simulink model "GreenCraneActualPrints"  (R2025b)
settings: Solver=VariableStepAuto  StartTime=0.0  StopTime=30  RelTol=1e-3
model workspace (MATLAB code in the model file):
  | clear;
  | %% Hydraulics
  | 
  | %Liquid
  | rho = 875;
  | beta = 1000; %MPa
  | 
  | %Pump
  | pP = 10e6; %100 bar i pascal, velger den sjøl med å skru
  | 
  | %Initial pA_Cyl
  | pA_Cyl_Initial = 67;    %Bar
  | 
  | %-------------------DCV-----------------------
  | dp0 = 20e5; %Nominal pressure drop, Pa
  | Q0 = 18/6e4; %Nominal flow, m^3/s
  | Cd = 0.55; %Discharge coefficient
  | AdMax_SI = Q0/(Cd*(2/rho*dp0)^0.5); %Discharge area m^2
  | AdMax = AdMax_SI*1e6;
  | 
  | Tau_DCV = 0.1; % [s] foreløbig
  | 
  | %TauP = 0.322; % Tau for pressure lowpass filter 49Hz veldig kraftig det fra Twincat
  | TauP = 1/(2*pi*5); % 5hz
  | %% DCV Orifice Area Vectors
  | 
  | % Deadband control signal thresholds
  | u_dead_up    = 0.236;
  | u_dead_down  = 0.206;
  | 
  | % Spool position at deadband
  | spool_dead_up   = 1.1182 * u_dead_up   - 0.0325;
  | spool_dead_down = 1.1075 * u_dead_down - 0.0416;
  | 
  | % Polynomial: spool position as function of Kv [L/min/sqrt(bar)]
  | % Valid from u = 0.25 to max stroke
  | p_spool_of_Kv_up   = [0.0018653, -0.033672,  0.22033, -0.65618,  0.83411, -0.047269, 0.26252];
  | p_spool_of_Kv_down = [0.00098272, -0.017507,  0.11599, -0.34851,  0.41222,  0.17643,  0.2076];
  | 
  | % Linear model slopes: spool_pos = spool_dead + slope * Kv
  | slope_Kv_up   = 0.3410;
  | slope_Kv_down = 0.4248;
  | 
  | % Evaluate polynomial over valid Kv range
  | Kv_range   = linspace(0.09, 4, 10000);
  | spool_up   = polyval(p_spool_of_Kv_up,   Kv_range);
  | spool_down = polyval(p_spool_of_Kv_down, Kv_range);
  | 
  | % Breakpoints: u = 0.25 to 0.50 in steps of 0.05, then max
  | u_breakpoints = 0.25:0.05:1.0;
  | 
  | % Corresponding spool positions
  | spool_bp_up   = 1.1182 * u_breakpoints - 0.0325;
  | spool_bp_down = 1.1075 * u_breakpoints - 0.0416;
  | 
  | % Find Kv at each breakpoint using nearest-index lookup
  | Kv_bp_up   = zeros(1, length(u_breakpoints));
  | Kv_bp_down = zeros(1, length(u_breakpoints));
  | for i = 1:length(u_breakpoints)
  |     if u_breakpoints(i) <= 0.25
  |         % Use linear model for transition point
  |         Kv_bp_up(i)   = (spool_bp_up(i)   - spool_dead_up)   / slope_Kv_up;
  |         Kv_bp_down(i) = (spool_bp_down(i) - spool_dead_down) / slope_Kv_down;
  |     else
  |         % Use polynomial inversion via nearest-index lookup
  |         [~, idx_up]   = min(abs(spool_up   - spool_bp_up(i)));
  |         [~, idx_down] = min(abs(spool_down - spool_bp_down(i)));
  |         Kv_bp_up(i)   = Kv_range(idx_up);
  |         Kv_bp_down(i) = Kv_range(idx_down);
  |     end
  | end
  | 
  | % Kv at max spool
  | [~, idx_max_up]   = max(spool_up);
  | [~, idx_max_down] = max(spool_down);
  | Kv_max_up   = Kv_range(idx_max_up);
  | Kv_max_down = Kv_range(idx_max_down);
  | 
  | % Unit conversion: L/min/sqrt(bar) -> m³/s/sqrt(Pa)
  | Kv_unit_conv = sqrt(1e-5) / 6e4;
  | 
  | % Convert all Kv breakpoints to area [m²]
  | A_bp_up   = (Kv_bp_up   * Kv_unit_conv) / (Cd * sqrt(2/rho));
  | A_bp_down = (Kv_bp_down * Kv_unit_conv) / (Cd * sqrt(2/rho));
  | A_max_up  = (Kv_max_up  * Kv_unit_conv) / (Cd * sqrt(2/rho));
  | A_max_down= (Kv_max_down* Kv_unit_conv) / (Cd * sqrt(2/rho));
  | 
  | % Orifice area vectors [m²]: [leakage, crack-open, u=0.30...0.50, fully-open]
  | orifice_area_up   = [1e-9, A_bp_up,   A_max_up];
  | orifice_area_down = [1e-9, A_bp_down, A_max_down];
  | 
  | % Control member position vectors (must match area vectors one-to-one)
  | u_max_pos = 1.05; % position for max area point, beyond valid range to avoid duplicate
  | % control_pos_up   = [0, u_breakpoints, u_max_pos];
  | % control_pos_down = [0, u_breakpoints, u_max_pos]; Nye under
  | 
  | control_pos_up   = [0, spool_bp_up,   1.1182 * u_max_pos - 0.0325];
  | control_pos_down = [0, spool_bp_down, 1.1075 * u_max_pos - 0.0416];
  | 
  | % ------------------CBV-------------------
  | alpha = 5; %Pilot ratio
  | pCr_A = 230e5; %Pa.
  | dp_open_A = 150e5; %Pa setter lik pcrack først
  | 
  | Cd_CBV = 0.8;
  | AdMax_CBV = (60 / 6e4) / sqrt(2/rho * 16e5) / Cd_CBV; %SJekk over denne
  | 
  | %-----------------Cylinder-----------------
  | d = 65; %mm
  | dr = 35; %mm
  | A = pi*d^2/4; %mm^2
  | Ar = pi*dr^2/4;  %mm^2
  | Aa = A - Ar; %mm^2
  | h = 500; %mm slaglengde
  | L0 = 272; %mm , dødlengde
  | dx = 0; %Dummy mm dx er mellom 0 og 500mm
  | L = h + L0 + dx; %mm variable length eller initial pos
  | 
  | %Weight (bruker ikke lenger?)
  | m = 75*4 + 20 + 90; %kg
  | g = 9.81; %m/s^2
  | MG = m*g; %Force from weight
  | 
  | %inital postition
  | x_Init = 100; %mm
  | 
  | 
  | %% Geometric properties
  | 
  | % Cylinder Translation lower hinge
  | Cx = 427; %mm translation from global coordinate
  | Cz = -1057; %mm translation
  | 
  | % Crane arm
  | theta_Init = 73.04- 90; %deg når kran er nede
  | thetaDot_Init = 0;
  | L1 = 3680; %mm length of beam
  | B1 = 100; %mm width of beam
  | H1 = 150; %mm height
  | t1 = 6; %mm thickness
  | revBasePinDia = 60; %mm of the pin in the main hinge
  | revBasePinLength = 185.5; %mm of the pin in the main hinge
  | 
  | %Cylinder
  | rEar = 35; %mm radius of the bearing ear
  | tEar = 30; %mm thickness of ear
  | earToCylTop = 52.45; %mm center of ear to top of cylinder in bottom pos
  | earToCylBot = 40.62; %mm center of ear to bottom cylinder in bottom pos
  | cylDia = 75; %mm Diameter of cylinger housing
  | cylLength = 682; %mm length of housing
  | rodLength = 565.26; %mm length of rod
  | rodDia = 35; %mm rod diameter
  | rodToCyl = 132; %mm Length in bottom pos from bottom of cylinder to bottom of rod without rod plate
  | revCylPinDia = 25; %mm diameter of the pin that the bearing of the top and bottom of cylinder revolves around
  | revCylPinLength = 84; %mm length of the pin
  | rPiston = 65/2; %mm radius of piston
  | tPiston = 40; %mm thickness of piston
  | 
  | %Ear top from global coordinate system
  | abx = 564.99; %mm; in the bottom pos
  | aby = 133; %mm in the bottom pos
  | 
  | % PayLoad
  | L2 = 210; %mm of the whole weight block
  | B2 = 700; %mm
  | H2 = 300; %mm
  | dY_PL_Beam = 75; %mm center of beam to center of payload
  | 
  | %% Mass properties (mass and center of mass)
  | beam_mass = 415.740; %kg mass of payload and beam
  | beam_COM = [3216.15, 61.48, 0.00]; %mm Old value x=3013.15mm
  | 
  | cyl_house_mass = 10.46699; %kg
  | cyl_house_COM = [260.99, 0.16, 0.00]; %mm from center of lowerjoint coordinate system
  | 
  | cyl_rod_mass = 4.81658; %kg mass of cylinder rod and piston
  | cyl_rod_COM = [-292.43, 0.00, 0.00]; %mm from upperjoint
  | %rod er feil
  | 
  | %% Inertia properties (Moments of inertia and products of inertia)
  | beam_MOI = [17.5673, 453.1288, 442.0275];   % kg·m^2 Mulig feil rekkefølge
  | beam_POI = [13.7279, 0.00000, 0.00000];  % kg·m^2
  | 
  | cyl_house_MOI = [0.00969, 0.50582, 0.50623]; %kgm^2
  | cyl_house_POI = [-0.00039, 0.00000, 0.00000]; % kgm^2
  | 
  | cyl_rod_MOI = [0.00142, 0.20919, 0.20942]; %kgm^2
  | cyl_rod_POI = [0.00000, 0.00000, 0.00000]; %kgm^2
  | 
  | 
  | % Er ganske sikker på at alle inertiaene er feil, basert på chat.
  | % At siden vi flytter oss til center of mass å må inertia være i henholdt til det.
  | 
  | %% Friction parameters
  | F_C   = 609;     % Coulomb friction force [N] 609 før
  | v_th  = 1e-3;    % Regularisation velocity threshold [m/s]
  | 
  | %% Pressure gradient feedback
  | 
  | dt = 0.001;     % timestep
  | TauF = 0.01;    % filter time constant in seconds.
  | Kf = 0.0005;     % Pressure feedback gain
undefined symbols (not defined in the file): orifice_area_up, X, Y, Z
libraries: sm_lib x41, fl_lib x19, nesl_utility x16, SimscapeFluids_lib x7, slpidlib x1
(part 1 of 2)
settings Model: Creator=michaerh  LastModifiedBy=sujro

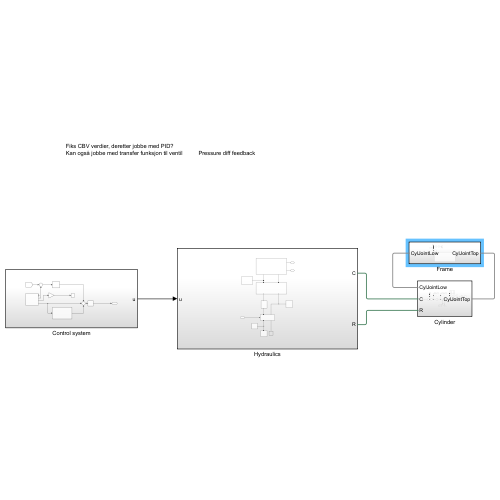
[thumbnail: Simulink's stored preview of the top-level diagram]
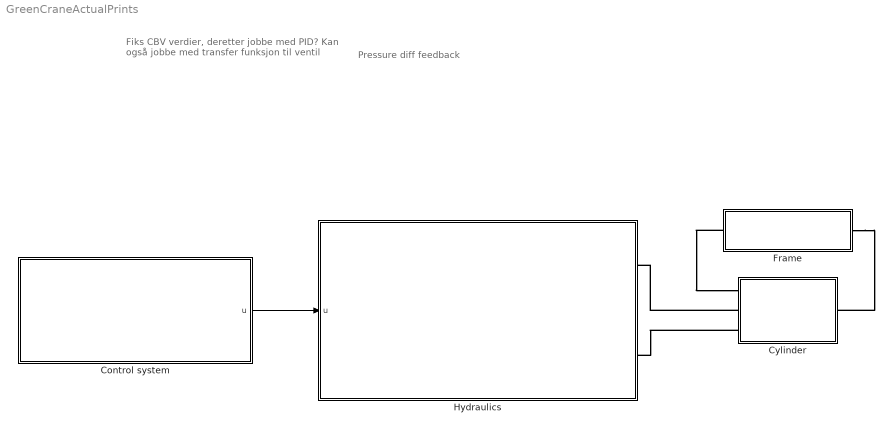
== system GreenCraneActualPrints ==
  note: Pressure diff feedback
  note: Fiks CBV verdier, deretter jobbe med PID?
      | Kan også jobbe med transfer funksjon til ventil
  Control system : Subsystem
  Cylinder : Subsystem
  Frame : Subsystem
  Hydraulics : Subsystem
  wires:
  Control system/1(u) -> Hydraulics/1(u)
  connections:
  Frame/RConn1 -- Cylinder/RConn1
  Frame/LConn1 -- Cylinder/LConn1
  Cylinder/LConn3 -- Hydraulics/RConn2
  Cylinder/LConn2 -- Hydraulics/RConn1

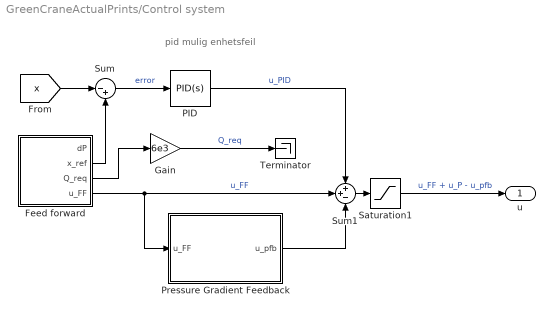
== system GreenCraneActualPrints/Control system ==
  note: pid mulig enhetsfeil
  Feed forward : Subsystem
  Gain : Gain  Gain=6e3
  PID : slpidlib/PID Controller  Controller=PID  Form=Parallel  TimeDomain=Continuous-time  UseExternalTs=off  SampleTime=-1  IntegratorMethod=Forward Euler  FilterMethod=Forward Euler  ControllerParametersSource=internal  P=8  I=0  UseKiTs=off  D=0  UseExternalDerivativeSource=off  N=100  UseFilter=on  TunerSelectOption=Transfer Function Based (PID Tuner App)  InitialConditionSource=internal  InitialConditionForIntegrator=0  InitialConditionForFilter=0  DifferentiatorICPrevScaledInput=0  ExternalReset=none  TrackingMode=off  Kt=1  LimitOutput=off  SatLimitsSource=internal  UpperSaturationLimit=inf  LowerSaturationLimit=-inf  LinearizeAsGain=on  AntiWindupMode=none  Kb=1  LimitIntegrator=off  UpperIntegratorSaturationLimit=inf  LowerIntegratorSaturationLimit=-inf  POutMin=[]  POutMax=[]  IOutMin=[]  IOutMax=[]  DOutMin=[]  DOutMax=[]  NOutMin=[]  NOutMax=[]  SumOutMin=[]  SumOutMax=[]  SaturationOutMin=[]  SaturationOutMax=[]  PParamMin=[]  PParamMax=[]  IParamMin=[]  IParamMax=[]  DParamMin=[]  DParamMax=[]  NParamMin=[]  NParamMax=[]  KbParamMin=[]  KbParamMax=[]  KtParamMin=[]  KtParamMax=[]  KbOutMin=[]  KbOutMax=[]  KtOutMin=[]  KtOutMax=[]  IntegratorOutMin=[]  IntegratorOutMax=[]  FilterOutMin=[]  FilterOutMax=[]  SumI1OutMin=[]  SumI1OutMax=[]  SumI2OutMin=[]  SumI2OutMax=[]  SumI3OutMin=[]  SumI3OutMax=[]  SumI4OutMin=[]  SumI4OutMax=[]  SumDOutMin=[]  SumDOutMax=[]  DifferentiatorOutMin=[]  DifferentiatorOutMax=[]  FilterDiffOutCoefMin=[]  FilterDiffOutCoefMax=[]  ReciprocalOutMin=[]  ReciprocalOutMax=[]  SumDenOutMin=[]  SumDenOutMax=[]  SumNumOutMin=[]  SumNumOutMax=[]  DivideOutMin=[]  DivideOutMax=[]  UdiffTsProdOutMin=[]  UdiffTsProdOutMax=[]  NTsProdOutMin=[]  NTsProdOutMax=[]  UintegralTsProdOutMin=[]  UintegralTsProdOutMax=[]  UngainTsProdOutMin=[]  UngainTsProdOutMax=[]  ClampingZeroOutDataTypeStr=Inherit: Inherit via back propagation  ClampingZeroOutMin=[]  ClampingZeroOutMax=[]  FilterDenConstantOutDataTypeStr=Inherit: Inherit via back propagation  FilterDenConstantOutMin=[]  FilterDenConstantOutMax=[]  PCopyOutDataTypeStr=Inherit: Inherit via back propagation  PCopyOutMin=[]  PCopyOutMax=[]  NCopyOutDataTypeStr=Inherit: Inherit via back propagation  NCopyOutMin=[]  NCopyOutMax=[]  IntegratorContinuousStateAttributes=''  IntegratorStateMustResolveToSignalObject=off  IntegratorRTWStateStorageClass=Auto  FilterContinuousStateAttributes=''  FilterStateMustResolveToSignalObject=off  FilterRTWStateStorageClass=Auto  ParallelPVariant=InternalParameters  IdealPVariant=Disabled  IVariant=InternalParameters  DVariant=InternalParameters  IntegratorVariant=Continuous  SatVariant=Disabled  AWVariant=Passthrough  PCopyVariant=Disabled  TRVariant=Disabled  FdbkBlocksVariant=Forward  IdealPFdbkVariant=Disabled  SatFdbkVariant=Disabled  DerivativeFilterVariant=ContFilter  NVariant=InternalParameters  NCopyVariant=Disabled  FilterICVariant=InternalICsFilter  IntegratorICVariant=InternalICs  ExternalResetVariant=Disabled  TRSumVariant=Passthrough  SumFdbkVariant=Disabled  SumVariant=Sum_PID  TsampFilterVariant=InternalTs  TsampNgainVariant=Passthrough  TsampIntegralVariant=Disabled_SignalSpec  ExternalSaturationOutDataTypeStr=Inherit: Same as second input  DerivativeSourceVariant=ErrorSignal  PreIntVariant=InternalPreInt
  Pressure Gradient Feedback : Subsystem
  Saturation1 : Saturate  UpperLimit=1  LowerLimit=-1
  Sum : Sum  Inputs=|-+
  Sum1 : Sum  Inputs=++-
  Terminator : Terminator
  u : Outport
  wires:
  [x] -> Sum/1
  Sum/1 -> PID/1  "error"
  Feed forward/3(Q_req) -> Gain/1
  Feed forward/2(x_ref) -> Sum/2
  Feed forward/4(u_FF) -> Pressure Gradient Feedback/1(u_FF), Sum1/2  "u_FF"
  Sum1/1 -> Saturation1/1
  Gain/1 -> Terminator/1  "Q_req"
  PID/1 -> Sum1/1  "u_PID"
  Saturation1/1 -> u/1  "u_FF + u_P - u_pfb"
  Pressure Gradient Feedback/1(u_pfb) -> Sum1/3

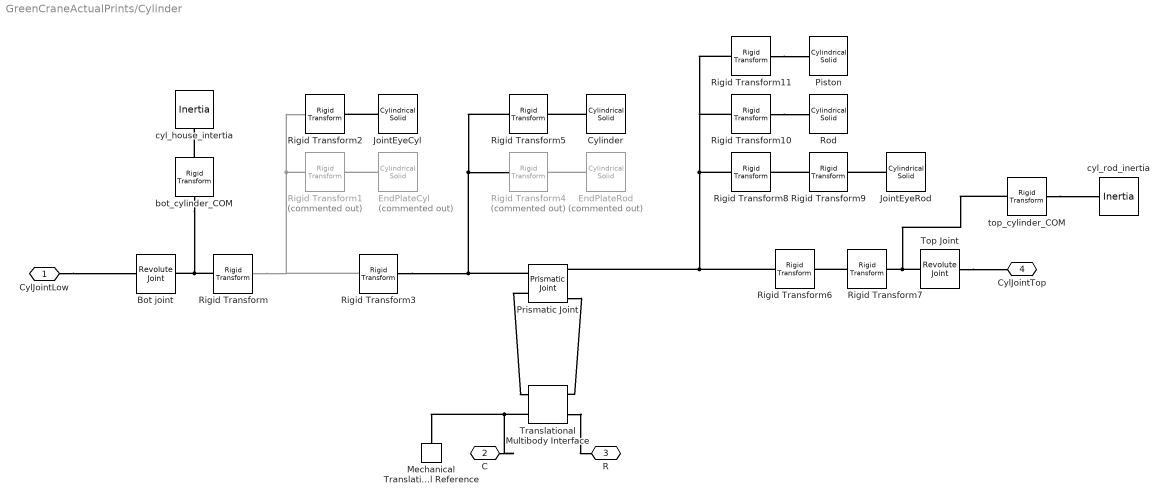
== system GreenCraneActualPrints/Cylinder ==
  Bot joint : sm_lib/Joints/Revolute Joint  JointMode=Normal  CompositeWrenchDir=FollowerOnBase  CompositeWrenchFrame=BaseFrame  SenseConstraintForce=off  SenseConstraintTorque=off  SenseTotalForce=off  SenseTotalTorque=off  PositionTargetSpecify=off  PositionTargetPriority=High  PositionTargetValue=0  PositionTargetValueUnits=deg  VelocityTargetSpecify=off  VelocityTargetPriority=High  VelocityTargetValue=0  VelocityTargetValueUnits=deg/s  EquilibriumPosition=0  EquilibriumPositionUnits=deg  SpringStiffness=0  SpringStiffnessUnits=N*m/deg  DampingCoefficient=0  DampingCoefficientUnits=N*m/(deg/s)  LowerLimitSpecify=off  LowerLimitBound=-90  LowerLimitBoundUnits=deg  LowerLimitStiffness=1e4  LowerLimitStiffnessUnits=N*m/deg  LowerLimitDamping=10  LowerLimitDampingUnits=N*m/(deg/s)  LowerLimitTransitionRegionWidth=0.1  LowerLimitTransitionRegionWidthUnits=deg  UpperLimitSpecify=off  UpperLimitBound=90  UpperLimitBoundUnits=deg  UpperLimitStiffness=1e4  UpperLimitStiffnessUnits=N*m/deg  UpperLimitDamping=10  UpperLimitDampingUnits=N*m/(deg/s)  UpperLimitTransitionRegionWidth=0.1  UpperLimitTransitionRegionWidthUnits=deg  TorqueActuationMode=NoTorque  MotionActuationMode=ComputedMotion  SensePosition=off  SenseVelocity=off  SenseAcceleration=off  SenseTorqueForce=off  SenseLowerLimitTorqueForce=off  SenseUpperLimitTorqueForce=off
  Cylinder : sm_lib/Body Elements/Cylindrical Solid  CylinderRadius=cylDia/2  CylinderRadiusUnits=mm  CylinderLength=cylLength  CylinderLengthUnits=mm  ExportEntireGeometry=off  InertiaType=Custom  BasedOnType=Density  Density=1000  DensityUnits=kg/m^3  Mass=1  MassUnits=kg  CenterOfMass=[0 0 0]  CenterOfMassUnits=m  MomentsOfInertia=[1 1 1]  MomentsOfInertiaUnits=kg*m^2  ProductsOfInertia=[0 0 0]  ProductsOfInertiaUnits=kg*m^2  GraphicType=FromGeometry  MarkerShape=Sphere  MarkerSize=10  GraphicVisPropType=SimpleVisualProperties  GraphicDiffuseColor=[0.3255 0.6863 1]  GraphicOpacity=1  GraphicSpecularColor=[0.5 0.5 0.5 1.0]  GraphicAmbientColor=[0.15 0.15 0.15 1.0]  GraphicEmissiveColor=[0.0 0.0 0.0 1.0]  GraphicShininess=75  DoExposeReferenceFrame=on  SerializedFrames=<Frames/>
  EndPlateCyl : sm_lib/Body Elements/Cylindrical Solid  Commented=on  CylinderRadius=0.040625  CylinderRadiusUnits=m  CylinderLength=0.066667  CylinderLengthUnits=m  ExportEntireGeometry=off  InertiaType=CalculateFromGeometry  BasedOnType=Density  Density=1000  DensityUnits=kg/m^3  Mass=1  MassUnits=kg  CenterOfMass=[0 0 0]  CenterOfMassUnits=m  MomentsOfInertia=[1 1 1]  MomentsOfInertiaUnits=kg*m^2  ProductsOfInertia=[0 0 0]  ProductsOfInertiaUnits=kg*m^2  GraphicType=FromGeometry  MarkerShape=Sphere  MarkerSize=10  GraphicVisPropType=SimpleVisualProperties  GraphicDiffuseColor=[0.5 0.5 0.5]  GraphicOpacity=1  GraphicSpecularColor=[0.5 0.5 0.5 1.0]  GraphicAmbientColor=[0.15 0.15 0.15 1.0]  GraphicEmissiveColor=[0.0 0.0 0.0 1.0]  GraphicShininess=75  DoExposeReferenceFrame=on  SerializedFrames=<Frames/>
  EndPlateRod : sm_lib/Body Elements/Cylindrical Solid  Commented=on  CylinderRadius=0.040625  CylinderRadiusUnits=m  CylinderLength=0.06667  CylinderLengthUnits=m  ExportEntireGeometry=off  InertiaType=CalculateFromGeometry  BasedOnType=Density  Density=1000  DensityUnits=kg/m^3  Mass=1  MassUnits=kg  CenterOfMass=[0 0 0]  CenterOfMassUnits=m  MomentsOfInertia=[1 1 1]  MomentsOfInertiaUnits=kg*m^2  ProductsOfInertia=[0 0 0]  ProductsOfInertiaUnits=kg*m^2  GraphicType=FromGeometry  MarkerShape=Sphere  MarkerSize=10  GraphicVisPropType=SimpleVisualProperties  GraphicDiffuseColor=[0.5 0.5 0.5]  GraphicOpacity=1  GraphicSpecularColor=[0.5 0.5 0.5 1.0]  GraphicAmbientColor=[0.15 0.15 0.15 1.0]  GraphicEmissiveColor=[0.0 0.0 0.0 1.0]  GraphicShininess=75  DoExposeReferenceFrame=on  SerializedFrames=<Frames/>
  JointEyeCyl : sm_lib/Body Elements/Cylindrical Solid  CylinderRadius=rEar  CylinderRadiusUnits=mm  CylinderLength=tEar  CylinderLengthUnits=mm  ExportEntireGeometry=off  InertiaType=Custom  BasedOnType=Density  Density=1000  DensityUnits=kg/m^3  Mass=1  MassUnits=kg  CenterOfMass=[0 0 0]  CenterOfMassUnits=m  MomentsOfInertia=[1 1 1]  MomentsOfInertiaUnits=kg*m^2  ProductsOfInertia=[0 0 0]  ProductsOfInertiaUnits=kg*m^2  GraphicType=FromGeometry  MarkerShape=Sphere  MarkerSize=10  GraphicVisPropType=SimpleVisualProperties  GraphicDiffuseColor=[0.7373 0.7373 0.7373]  GraphicOpacity=1  GraphicSpecularColor=[0.5 0.5 0.5 1.0]  GraphicAmbientColor=[0.15 0.15 0.15 1.0]  GraphicEmissiveColor=[0.0 0.0 0.0 1.0]  GraphicShininess=75  DoExposeReferenceFrame=on  SerializedFrames=<Frames/>
  JointEyeRod : sm_lib/Body Elements/Cylindrical Solid  CylinderRadius=rEar  CylinderRadiusUnits=mm  CylinderLength=tEar  CylinderLengthUnits=mm  ExportEntireGeometry=off  InertiaType=Custom  BasedOnType=Density  Density=1000  DensityUnits=kg/m^3  Mass=1  MassUnits=kg  CenterOfMass=[0 0 0]  CenterOfMassUnits=m  MomentsOfInertia=[1 1 1]  MomentsOfInertiaUnits=kg*m^2  ProductsOfInertia=[0 0 0]  ProductsOfInertiaUnits=kg*m^2  GraphicType=FromGeometry  MarkerShape=Sphere  MarkerSize=10  GraphicVisPropType=SimpleVisualProperties  GraphicDiffuseColor=[0.7373 0.7373 0.7373]  GraphicOpacity=1  GraphicSpecularColor=[0.5 0.5 0.5 1.0]  GraphicAmbientColor=[0.15 0.15 0.15 1.0]  GraphicEmissiveColor=[0.0 0.0 0.0 1.0]  GraphicShininess=75  DoExposeReferenceFrame=on  SerializedFrames=<Frames/>
  Mechanical Translational Reference : fl_lib/Mechanical/Translational Elements/Mechanical Translational Reference
  Piston : sm_lib/Body Elements/Cylindrical Solid  CylinderRadius=rPiston  CylinderRadiusUnits=mm  CylinderLength=tPiston  CylinderLengthUnits=mm  ExportEntireGeometry=off  InertiaType=Custom  BasedOnType=Density  Density=1000  DensityUnits=kg/m^3  Mass=0.1  MassUnits=kg  CenterOfMass=[0 0 0]  CenterOfMassUnits=m  MomentsOfInertia=[1 1 1]  MomentsOfInertiaUnits=kg*m^2  ProductsOfInertia=[0 0 0]  ProductsOfInertiaUnits=kg*m^2  GraphicType=FromGeometry  MarkerShape=Sphere  MarkerSize=10  GraphicVisPropType=SimpleVisualProperties  GraphicDiffuseColor=[0.2314 0.2314 0.2314]  GraphicOpacity=1  GraphicSpecularColor=[0.5 0.5 0.5 1.0]  GraphicAmbientColor=[0.15 0.15 0.15 1.0]  GraphicEmissiveColor=[0.0 0.0 0.0 1.0]  GraphicShininess=75  DoExposeReferenceFrame=on  SerializedFrames=<Frames/>
  Prismatic Joint : sm_lib/Joints/Prismatic Joint  JointMode=Normal  CompositeWrenchDir=FollowerOnBase  CompositeWrenchFrame=BaseFrame  SenseConstraintForce=off  SenseConstraintTorque=off  SenseTotalForce=off  SenseTotalTorque=off  PositionTargetSpecify=off  PositionTargetPriority=Low  PositionTargetValue=x_Init  PositionTargetValueUnits=mm  VelocityTargetSpecify=on  VelocityTargetPriority=High  VelocityTargetValue=0  VelocityTargetValueUnits=m/s  EquilibriumPosition=0  EquilibriumPositionUnits=m  SpringStiffness=0  SpringStiffnessUnits=N/m  DampingCoefficient=0  DampingCoefficientUnits=N/(m/s)  LowerLimitSpecify=off  LowerLimitBound=-1  LowerLimitBoundUnits=m  LowerLimitStiffness=1e6  LowerLimitStiffnessUnits=N/m  LowerLimitDamping=1e3  LowerLimitDampingUnits=N/(m/s)  LowerLimitTransitionRegionWidth=1e-4  LowerLimitTransitionRegionWidthUnits=m  UpperLimitSpecify=off  UpperLimitBound=1  UpperLimitBoundUnits=m  UpperLimitStiffness=1e6  UpperLimitStiffnessUnits=N/m  UpperLimitDamping=1e3  UpperLimitDampingUnits=N/(m/s)  UpperLimitTransitionRegionWidth=1e-4  UpperLimitTransitionRegionWidthUnits=m  TorqueActuationMode=InputTorque  MotionActuationMode=ComputedMotion  SensePosition=on  SenseVelocity=on  SenseAcceleration=off  SenseTorqueForce=off  SenseLowerLimitTorqueForce=off  SenseUpperLimitTorqueForce=off
  Rigid Transform : sm_lib/Frames and Transforms/Rigid Transform  RotationMethod=RotationSequence  FollAlignAxisA=+X  BaseAlignAxisA=+Y  FollAlignAxisB=+Y  BaseAlignAxisB=+Z  RotationStandardAxis=+Z  RotationAngle=0  RotationAngleUnits=deg  RotationArbitraryAxis=[0 0 1]  RotationSequenceAxes=FollowerAxes  RotationSequence=XYX  RotationSequenceAngles=[0 90 0]  RotationSequenceAnglesUnits=deg  RotationMatrix=[1 0 0;0 1 0;0 0 1]  Quaternion=[1 0 0 0]  TranslationMethod=None  TranslationCartesianOffset=[0 0 0]  TranslationCartesianOffsetUnits=m  TranslationStandardAxis=+Z  TranslationStandardOffset=0  TranslationStandardOffsetUnits=m  TranslationROffset=0  TranslationROffsetUnits=m  TranslationThetaOffset=0  TranslationThetaOffsetUnits=deg  TranslationZOffset=0  TranslationZOffsetUnits=m
  Rigid Transform1 : sm_lib/Frames and Transforms/Rigid Transform  Commented=on  RotationMethod=None  FollAlignAxisA=+X  BaseAlignAxisA=+Y  FollAlignAxisB=+Y  BaseAlignAxisB=+Z  RotationStandardAxis=+Z  RotationAngle=0  RotationAngleUnits=deg  RotationArbitraryAxis=[0 0 1]  RotationSequenceAxes=FollowerAxes  RotationSequence=XYX  RotationSequenceAngles=[0 0 0]  RotationSequenceAnglesUnits=deg  RotationMatrix=[1 0 0;0 1 0;0 0 1]  Quaternion=[1 0 0 0]  TranslationMethod=Cartesian  TranslationCartesianOffset=[0 0 0.1]  TranslationCartesianOffsetUnits=m  TranslationStandardAxis=+Z  TranslationStandardOffset=0  TranslationStandardOffsetUnits=m  TranslationROffset=0  TranslationROffsetUnits=m  TranslationThetaOffset=0  TranslationThetaOffsetUnits=deg  TranslationZOffset=0  TranslationZOffsetUnits=m
  Rigid Transform10 : sm_lib/Frames and Transforms/Rigid Transform  RotationMethod=None  FollAlignAxisA=+X  BaseAlignAxisA=+Y  FollAlignAxisB=+Y  BaseAlignAxisB=+Z  RotationStandardAxis=+Z  RotationAngle=0  RotationAngleUnits=deg  RotationArbitraryAxis=[0 0 1]  RotationSequenceAxes=FollowerAxes  RotationSequence=XYX  RotationSequenceAngles=[0 0 0]  RotationSequenceAnglesUnits=deg  RotationMatrix=[1 0 0;0 1 0;0 0 1]  Quaternion=[1 0 0 0]  TranslationMethod=Cartesian  TranslationCartesianOffset=[0,0,rodLength/2 + rodToCyl]  TranslationCartesianOffsetUnits=mm  TranslationStandardAxis=+Z  TranslationStandardOffset=0  TranslationStandardOffsetUnits=m  TranslationROffset=0  TranslationROffsetUnits=m  TranslationThetaOffset=0  TranslationThetaOffsetUnits=deg  TranslationZOffset=0  TranslationZOffsetUnits=m
  Rigid Transform11 : sm_lib/Frames and Transforms/Rigid Transform  RotationMethod=None  FollAlignAxisA=+X  BaseAlignAxisA=+Y  FollAlignAxisB=+Y  BaseAlignAxisB=+Z  RotationStandardAxis=+Z  RotationAngle=0  RotationAngleUnits=deg  RotationArbitraryAxis=[0 0 1]  RotationSequenceAxes=FollowerAxes  RotationSequence=XYX  RotationSequenceAngles=[0 0 0]  RotationSequenceAnglesUnits=deg  RotationMatrix=[1 0 0;0 1 0;0 0 1]  Quaternion=[1 0 0 0]  TranslationMethod=Cartesian  TranslationCartesianOffset=[0,0,rodToCyl + tPiston/2]  TranslationCartesianOffsetUnits=mm  TranslationStandardAxis=+Z  TranslationStandardOffset=0  TranslationStandardOffsetUnits=m  TranslationROffset=0  TranslationROffsetUnits=m  TranslationThetaOffset=0  TranslationThetaOffsetUnits=deg  TranslationZOffset=0  TranslationZOffsetUnits=m
  Rigid Transform2 : sm_lib/Frames and Transforms/Rigid Transform  RotationMethod=RotationSequence  FollAlignAxisA=+X  BaseAlignAxisA=+Y  FollAlignAxisB=+Y  BaseAlignAxisB=+Z  RotationStandardAxis=+Z  RotationAngle=0  RotationAngleUnits=deg  RotationArbitraryAxis=[0 0 1]  RotationSequenceAxes=FollowerAxes  RotationSequence=XYZ  RotationSequenceAngles=[0 -90 0]  RotationSequenceAnglesUnits=deg  RotationMatrix=[1 0 0;0 1 0;0 0 1]  Quaternion=[1 0 0 0]  TranslationMethod=None  TranslationCartesianOffset=[0 0 0]  TranslationCartesianOffsetUnits=m  TranslationStandardAxis=+Z  TranslationStandardOffset=0  TranslationStandardOffsetUnits=m  TranslationROffset=0  TranslationROffsetUnits=m  TranslationThetaOffset=0  TranslationThetaOffsetUnits=deg  TranslationZOffset=0  TranslationZOffsetUnits=m
  Rigid Transform3 : sm_lib/Frames and Transforms/Rigid Transform  RotationMethod=None  FollAlignAxisA=+X  BaseAlignAxisA=+Y  FollAlignAxisB=+Y  BaseAlignAxisB=+Z  RotationStandardAxis=+Z  RotationAngle=0  RotationAngleUnits=deg  RotationArbitraryAxis=[0 0 1]  RotationSequenceAxes=FollowerAxes  RotationSequence=XYX  RotationSequenceAngles=[0 0 0]  RotationSequenceAnglesUnits=deg  RotationMatrix=[1 0 0;0 1 0;0 0 1]  Quaternion=[1 0 0 0]  TranslationMethod=Cartesian  TranslationCartesianOffset=[0 0 earToCylBot]  TranslationCartesianOffsetUnits=mm  TranslationStandardAxis=+Z  TranslationStandardOffset=0  TranslationStandardOffsetUnits=m  TranslationROffset=0  TranslationROffsetUnits=m  TranslationThetaOffset=0  TranslationThetaOffsetUnits=deg  TranslationZOffset=0  TranslationZOffsetUnits=m
  Rigid Transform4 : sm_lib/Frames and Transforms/Rigid Transform  Commented=on  RotationMethod=None  FollAlignAxisA=+X  BaseAlignAxisA=+Y  FollAlignAxisB=+Y  BaseAlignAxisB=+Z  RotationStandardAxis=+Z  RotationAngle=0  RotationAngleUnits=deg  RotationArbitraryAxis=[0 0 1]  RotationSequenceAxes=FollowerAxes  RotationSequence=XYX  RotationSequenceAngles=[0 0 0]  RotationSequenceAnglesUnits=deg  RotationMatrix=[1 0 0;0 1 0;0 0 1]  Quaternion=[1 0 0 0]  TranslationMethod=Cartesian  TranslationCartesianOffset=[0 0 0.61667]  TranslationCartesianOffsetUnits=m  TranslationStandardAxis=+Z  TranslationStandardOffset=0  TranslationStandardOffsetUnits=m  TranslationROffset=0  TranslationROffsetUnits=m  TranslationThetaOffset=0  TranslationThetaOffsetUnits=deg  TranslationZOffset=0  TranslationZOffsetUnits=m
  Rigid Transform5 : sm_lib/Frames and Transforms/Rigid Transform  RotationMethod=None  FollAlignAxisA=+X  BaseAlignAxisA=+Y  FollAlignAxisB=+Y  BaseAlignAxisB=+Z  RotationStandardAxis=+Z  RotationAngle=0  RotationAngleUnits=deg  RotationArbitraryAxis=[0 0 1]  RotationSequenceAxes=FollowerAxes  RotationSequence=XYX  RotationSequenceAngles=[0 0 0]  RotationSequenceAnglesUnits=deg  RotationMatrix=[1 0 0;0 1 0;0 0 1]  Quaternion=[1 0 0 0]  TranslationMethod=Cartesian  TranslationCartesianOffset=[0 0 cylLength/2]  TranslationCartesianOffsetUnits=mm  TranslationStandardAxis=+Z  TranslationStandardOffset=0  TranslationStandardOffsetUnits=m  TranslationROffset=0  TranslationROffsetUnits=m  TranslationThetaOffset=0  TranslationThetaOffsetUnits=deg  TranslationZOffset=0  TranslationZOffsetUnits=m
  Rigid Transform6 : sm_lib/Frames and Transforms/Rigid Transform  RotationMethod=None  FollAlignAxisA=+X  BaseAlignAxisA=+Y  FollAlignAxisB=+Y  BaseAlignAxisB=+Z  RotationStandardAxis=+Z  RotationAngle=0  RotationAngleUnits=deg  RotationArbitraryAxis=[0 0 1]  RotationSequenceAxes=FollowerAxes  RotationSequence=XYX  RotationSequenceAngles=[0 0 0]  RotationSequenceAnglesUnits=deg  RotationMatrix=[1 0 0;0 1 0;0 0 1]  Quaternion=[1 0 0 0]  TranslationMethod=Cartesian  TranslationCartesianOffset=[0 0 cylLength + earToCylTop]  TranslationCartesianOffsetUnits=mm  TranslationStandardAxis=+Z  TranslationStandardOffset=0  TranslationStandardOffsetUnits=m  TranslationROffset=0  TranslationROffsetUnits=m  TranslationThetaOffset=0  TranslationThetaOffsetUnits=deg  TranslationZOffset=0  TranslationZOffsetUnits=m
  Rigid Transform7 : sm_lib/Frames and Transforms/Rigid Transform  RotationMethod=RotationSequence  FollAlignAxisA=+X  BaseAlignAxisA=+Y  FollAlignAxisB=+Y  BaseAlignAxisB=+Z  RotationStandardAxis=+Z  RotationAngle=0  RotationAngleUnits=deg  RotationArbitraryAxis=[0 0 1]  RotationSequenceAxes=FollowerAxes  RotationSequence=XYZ  RotationSequenceAngles=[0 -90 0]  RotationSequenceAnglesUnits=deg  RotationMatrix=[1 0 0;0 1 0;0 0 1]  Quaternion=[1 0 0 0]  TranslationMethod=None  TranslationCartesianOffset=[0 0 0]  TranslationCartesianOffsetUnits=m  TranslationStandardAxis=+Z  TranslationStandardOffset=0  TranslationStandardOffsetUnits=m  TranslationROffset=0  TranslationROffsetUnits=m  TranslationThetaOffset=0  TranslationThetaOffsetUnits=deg  TranslationZOffset=0  TranslationZOffsetUnits=m
  Rigid Transform8 : sm_lib/Frames and Transforms/Rigid Transform  RotationMethod=None  FollAlignAxisA=+X  BaseAlignAxisA=+Y  FollAlignAxisB=+Y  BaseAlignAxisB=+Z  RotationStandardAxis=+Z  RotationAngle=0  RotationAngleUnits=deg  RotationArbitraryAxis=[0 0 1]  RotationSequenceAxes=FollowerAxes  RotationSequence=XYX  RotationSequenceAngles=[0 0 0]  RotationSequenceAnglesUnits=deg  RotationMatrix=[1 0 0;0 1 0;0 0 1]  Quaternion=[1 0 0 0]  TranslationMethod=Cartesian  TranslationCartesianOffset=[0,0,cylLength+ earToCylTop]  TranslationCartesianOffsetUnits=mm  TranslationStandardAxis=+Z  TranslationStandardOffset=0  TranslationStandardOffsetUnits=m  TranslationROffset=0  TranslationROffsetUnits=m  TranslationThetaOffset=0  TranslationThetaOffsetUnits=deg  TranslationZOffset=0  TranslationZOffsetUnits=m
  Rigid Transform9 : sm_lib/Frames and Transforms/Rigid Transform  RotationMethod=RotationSequence  FollAlignAxisA=+X  BaseAlignAxisA=+Y  FollAlignAxisB=+Y  BaseAlignAxisB=+Z  RotationStandardAxis=+Z  RotationAngle=0  RotationAngleUnits=deg  RotationArbitraryAxis=[0 0 1]  RotationSequenceAxes=FollowerAxes  RotationSequence=XYZ  RotationSequenceAngles=[0 -90 0]  RotationSequenceAnglesUnits=deg  RotationMatrix=[1 0 0;0 1 0;0 0 1]  Quaternion=[1 0 0 0]  TranslationMethod=None  TranslationCartesianOffset=[0 0 0]  TranslationCartesianOffsetUnits=m  TranslationStandardAxis=+Z  TranslationStandardOffset=0  TranslationStandardOffsetUnits=m  TranslationROffset=0  TranslationROffsetUnits=m  TranslationThetaOffset=0  TranslationThetaOffsetUnits=deg  TranslationZOffset=0  TranslationZOffsetUnits=m
  Rod : sm_lib/Body Elements/Cylindrical Solid  CylinderRadius=rodDia/2  CylinderRadiusUnits=mm  CylinderLength=rodLength  CylinderLengthUnits=mm  ExportEntireGeometry=off  InertiaType=Custom  BasedOnType=Density  Density=1000  DensityUnits=kg/m^3  Mass=1  MassUnits=kg  CenterOfMass=[0 0 0]  CenterOfMassUnits=m  MomentsOfInertia=[1 1 1]  MomentsOfInertiaUnits=kg*m^2  ProductsOfInertia=[0 0 0]  ProductsOfInertiaUnits=kg*m^2  GraphicType=FromGeometry  MarkerShape=Sphere  MarkerSize=10  GraphicVisPropType=SimpleVisualProperties  GraphicDiffuseColor=[0.9137 0.9137 0.9137]  GraphicOpacity=1  GraphicSpecularColor=[0.5 0.5 0.5 1.0]  GraphicAmbientColor=[0.15 0.15 0.15 1.0]  GraphicEmissiveColor=[0.0 0.0 0.0 1.0]  GraphicShininess=75  DoExposeReferenceFrame=on  SerializedFrames=<Frames/>
  Top Joint : sm_lib/Joints/Revolute Joint  JointMode=Normal  CompositeWrenchDir=FollowerOnBase  CompositeWrenchFrame=BaseFrame  SenseConstraintForce=off  SenseConstraintTorque=off  SenseTotalForce=off  SenseTotalTorque=off  PositionTargetSpecify=off  PositionTargetPriority=High  PositionTargetValue=0  PositionTargetValueUnits=deg  VelocityTargetSpecify=off  VelocityTargetPriority=High  VelocityTargetValue=0  VelocityTargetValueUnits=deg/s  EquilibriumPosition=0  EquilibriumPositionUnits=deg  SpringStiffness=0  SpringStiffnessUnits=N*m/deg  DampingCoefficient=0  DampingCoefficientUnits=N*m/(deg/s)  LowerLimitSpecify=off  LowerLimitBound=-90  LowerLimitBoundUnits=deg  LowerLimitStiffness=1e4  LowerLimitStiffnessUnits=N*m/deg  LowerLimitDamping=10  LowerLimitDampingUnits=N*m/(deg/s)  LowerLimitTransitionRegionWidth=0.1  LowerLimitTransitionRegionWidthUnits=deg  UpperLimitSpecify=off  UpperLimitBound=90  UpperLimitBoundUnits=deg  UpperLimitStiffness=1e4  UpperLimitStiffnessUnits=N*m/deg  UpperLimitDamping=10  UpperLimitDampingUnits=N*m/(deg/s)  UpperLimitTransitionRegionWidth=0.1  UpperLimitTransitionRegionWidthUnits=deg  TorqueActuationMode=NoTorque  MotionActuationMode=ComputedMotion  SensePosition=off  SenseVelocity=off  SenseAcceleration=off  SenseTorqueForce=off  SenseLowerLimitTorqueForce=off  SenseUpperLimitTorqueForce=off
  Translational Multibody Interface : fl_lib/Mechanical/Multibody Interfaces/Translational Multibody Interface
  bot_cylinder_COM : sm_lib/Frames and Transforms/Rigid Transform  RotationMethod=None  FollAlignAxisA=+X  BaseAlignAxisA=+Y  FollAlignAxisB=+Y  BaseAlignAxisB=+Z  RotationStandardAxis=+Z  RotationAngle=0  RotationAngleUnits=deg  RotationArbitraryAxis=[0 0 1]  RotationSequenceAxes=FollowerAxes  RotationSequence=XYX  RotationSequenceAngles=[0 0 0]  RotationSequenceAnglesUnits=deg  RotationMatrix=[1 0 0;0 1 0;0 0 1]  Quaternion=[1 0 0 0]  TranslationMethod=Cartesian  TranslationCartesianOffset=cyl_house_COM  TranslationCartesianOffsetUnits=mm  TranslationStandardAxis=+Z  TranslationStandardOffset=0  TranslationStandardOffsetUnits=m  TranslationROffset=0  TranslationROffsetUnits=m  TranslationThetaOffset=0  TranslationThetaOffsetUnits=deg  TranslationZOffset=0  TranslationZOffsetUnits=m
  cyl_house_intertia : sm_lib/Body Elements/Inertia  InertiaType=Custom  Mass=1  MassUnits=kg  CenterOfMass=[0 0 0]  CenterOfMassUnits=m  MomentsOfInertia=cyl_house_MOI  MomentsOfInertiaUnits=kg*m^2  ProductsOfInertia=cyl_house_MOI  ProductsOfInertiaUnits=kg*m^2  GraphicType=Marker  MarkerShape=Inertia  MarkerSize=20  GraphicVisPropType=SimpleVisualProperties  GraphicDiffuseColor=[0.5 0.5 0.5]  GraphicOpacity=1  GraphicSpecularColor=[0.5 0.5 0.5 1.0]  GraphicAmbientColor=[0.15 0.15 0.15 1.0]  GraphicEmissiveColor=[0.0 0.0 0.0 1.0]  GraphicShininess=75
  cyl_rod_inertia : sm_lib/Body Elements/Inertia  InertiaType=Custom  Mass=1  MassUnits=kg  CenterOfMass=[0 0 0]  CenterOfMassUnits=m  MomentsOfInertia=cyl_rod_MOI  MomentsOfInertiaUnits=kg*m^2  ProductsOfInertia=cyl_rod_POI  ProductsOfInertiaUnits=kg*m^2  GraphicType=Marker  MarkerShape=Inertia  MarkerSize=20  GraphicVisPropType=SimpleVisualProperties  GraphicDiffuseColor=[0.5 0.5 0.5]  GraphicOpacity=1  GraphicSpecularColor=[0.5 0.5 0.5 1.0]  GraphicAmbientColor=[0.15 0.15 0.15 1.0]  GraphicEmissiveColor=[0.0 0.0 0.0 1.0]  GraphicShininess=75
  top_cylinder_COM : sm_lib/Frames and Transforms/Rigid Transform  RotationMethod=None  FollAlignAxisA=+X  BaseAlignAxisA=+Y  FollAlignAxisB=+Y  BaseAlignAxisB=+Z  RotationStandardAxis=+Z  RotationAngle=0  RotationAngleUnits=deg  RotationArbitraryAxis=[0 0 1]  RotationSequenceAxes=FollowerAxes  RotationSequence=XYX  RotationSequenceAngles=[0 0 0]  RotationSequenceAnglesUnits=deg  RotationMatrix=[1 0 0;0 1 0;0 0 1]  Quaternion=[1 0 0 0]  TranslationMethod=Cartesian  TranslationCartesianOffset=cyl_rod_COM  TranslationCartesianOffsetUnits=mm  TranslationStandardAxis=+Z  TranslationStandardOffset=0  TranslationStandardOffsetUnits=m  TranslationROffset=0  TranslationROffsetUnits=m  TranslationThetaOffset=0  TranslationThetaOffsetUnits=deg  TranslationZOffset=0  TranslationZOffsetUnits=m
  CylJointLow : PMIOPort  Side=Left
  C : PMIOPort  Port=2  Side=Left
  R : PMIOPort  Port=3  Side=Left
  CylJointTop : PMIOPort  Port=4  Side=Right
  connections:
  Rigid Transform/LConn1 -- bot_cylinder_COM/LConn1 -- Bot joint/RConn1
  CylJointLow/RConn1 -- Bot joint/LConn1
  Rigid Transform1/LConn1 -- Rigid Transform/RConn1 -- Rigid Transform3/LConn1 -- Rigid Transform2/LConn1
  EndPlateCyl/RConn1 -- Rigid Transform1/RConn1
  JointEyeCyl/RConn1 -- Rigid Transform2/RConn1
  Rigid Transform3/RConn1 -- Prismatic Joint/LConn1 -- Rigid Transform5/LConn1 -- Rigid Transform4/LConn1
  Cylinder/RConn1 -- Rigid Transform5/RConn1
  EndPlateRod/RConn1 -- Rigid Transform4/RConn1
  Prismatic Joint/LConn2 -- Translational Multibody Interface/LConn1
  Prismatic Joint/RConn3 -- Translational Multibody Interface/RConn1
  Rigid Transform6/LConn1 -- Rigid Transform11/LConn1 -- Rigid Transform10/LConn1 -- Rigid Transform8/LConn1 -- Prismatic Joint/RConn1
  Rigid Transform7/LConn1 -- Rigid Transform6/RConn1
  Top Joint/LConn1 -- top_cylinder_COM/LConn1 -- Rigid Transform7/RConn1
  Rigid Transform9/LConn1 -- Rigid Transform8/RConn1
  JointEyeRod/RConn1 -- Rigid Transform9/RConn1
  Rigid Transform10/RConn1 -- Rod/RConn1
  Rigid Transform11/RConn1 -- Piston/RConn1
  Translational Multibody Interface/LConn2 -- C/RConn1 -- Mechanical Translational Reference/LConn1
  Translational Multibody Interface/RConn2 -- R/RConn1
  Top Joint/RConn1 -- CylJointTop/RConn1
  top_cylinder_COM/RConn1 -- cyl_rod_inertia/RConn1
  bot_cylinder_COM/RConn1 -- cyl_house_intertia/RConn1

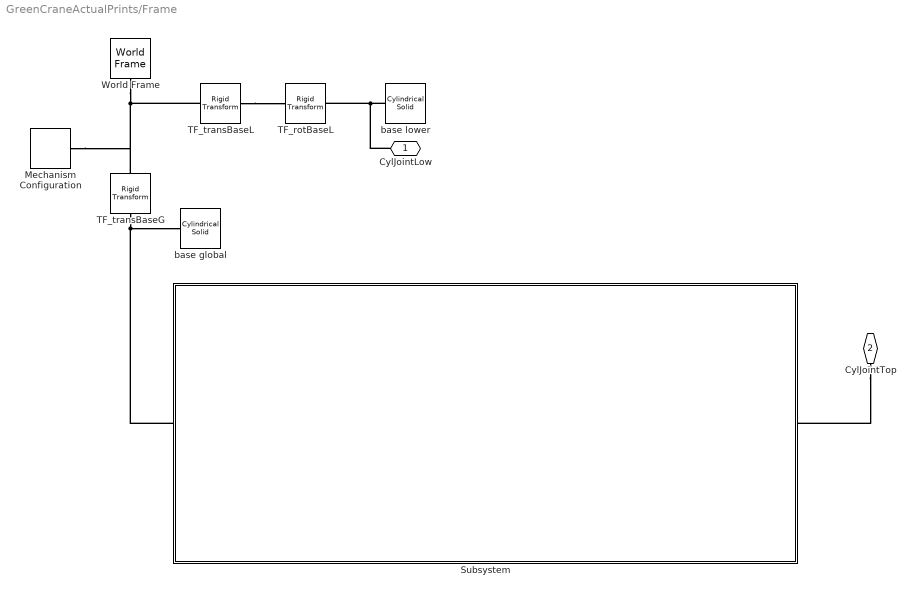
== system GreenCraneActualPrints/Frame ==
  Mechanism Configuration : sm_lib/Utilities/Mechanism Configuration  UniformGravity=Constant  GravityVector=[0 0 -9.80665]  GravityVectorUnits=m/s^2  LinearizationDelta=0.001  JointModeTransitionNonlinearIterations=2
  Subsystem : Subsystem
  TF_rotBaseL : sm_lib/Frames and Transforms/Rigid Transform  RotationMethod=RotationSequence  FollAlignAxisA=+X  BaseAlignAxisA=+Y  FollAlignAxisB=+Y  BaseAlignAxisB=+Z  RotationStandardAxis=+Z  RotationAngle=0  RotationAngleUnits=deg  RotationArbitraryAxis=[0 0 1]  RotationSequenceAxes=FollowerAxes  RotationSequence=XYZ  RotationSequenceAngles=[90 0 0]  RotationSequenceAnglesUnits=deg  RotationMatrix=[1 0 0;0 1 0;0 0 1]  Quaternion=[1 0 0 0]  TranslationMethod=Cartesian  TranslationCartesianOffset=[0 0 0]  TranslationCartesianOffsetUnits=m  TranslationStandardAxis=+Z  TranslationStandardOffset=0  TranslationStandardOffsetUnits=m  TranslationROffset=0  TranslationROffsetUnits=m  TranslationThetaOffset=0  TranslationThetaOffsetUnits=deg  TranslationZOffset=0  TranslationZOffsetUnits=m
  TF_transBaseG : sm_lib/Frames and Transforms/Rigid Transform  RotationMethod=RotationSequence  FollAlignAxisA=+X  BaseAlignAxisA=+Y  FollAlignAxisB=+Y  BaseAlignAxisB=+Z  RotationStandardAxis=+Z  RotationAngle=0  RotationAngleUnits=deg  RotationArbitraryAxis=[0 0 1]  RotationSequenceAxes=FollowerAxes  RotationSequence=XYZ  RotationSequenceAngles=[90 0 0]  RotationSequenceAnglesUnits=deg  RotationMatrix=[1 0 0;0 1 0;0 0 1]  Quaternion=[1 0 0 0]  TranslationMethod=Cartesian  TranslationCartesianOffset=[0 0 0]  TranslationCartesianOffsetUnits=m  TranslationStandardAxis=+Z  TranslationStandardOffset=0  TranslationStandardOffsetUnits=m  TranslationROffset=0  TranslationROffsetUnits=m  TranslationThetaOffset=0  TranslationThetaOffsetUnits=deg  TranslationZOffset=0  TranslationZOffsetUnits=m
  TF_transBaseL : sm_lib/Frames and Transforms/Rigid Transform  RotationMethod=None  FollAlignAxisA=+X  BaseAlignAxisA=+Y  FollAlignAxisB=+Y  BaseAlignAxisB=+Z  RotationStandardAxis=+Z  RotationAngle=0  RotationAngleUnits=deg  RotationArbitraryAxis=[0 0 1]  RotationSequenceAxes=FollowerAxes  RotationSequence=XYX  RotationSequenceAngles=[0 0 0]  RotationSequenceAnglesUnits=deg  RotationMatrix=[1 0 0;0 1 0;0 0 1]  Quaternion=[1 0 0 0]  TranslationMethod=Cartesian  TranslationCartesianOffset=[Cx 0 Cz]  TranslationCartesianOffsetUnits=mm  TranslationStandardAxis=+Z  TranslationStandardOffset=0  TranslationStandardOffsetUnits=m  TranslationROffset=0  TranslationROffsetUnits=m  TranslationThetaOffset=0  TranslationThetaOffsetUnits=deg  TranslationZOffset=0  TranslationZOffsetUnits=m
  World Frame : sm_lib/Frames and Transforms/World Frame
  base global : sm_lib/Body Elements/Cylindrical Solid  CylinderRadius=revBasePinDia/2  CylinderRadiusUnits=mm  CylinderLength=revBasePinLength  CylinderLengthUnits=mm  ExportEntireGeometry=off  InertiaType=CalculateFromGeometry  BasedOnType=Density  Density=1000  DensityUnits=kg/m^3  Mass=1  MassUnits=kg  CenterOfMass=[0 0 0]  CenterOfMassUnits=m  MomentsOfInertia=[1 1 1]  MomentsOfInertiaUnits=kg*m^2  ProductsOfInertia=[0 0 0]  ProductsOfInertiaUnits=kg*m^2  GraphicType=FromGeometry  MarkerShape=Sphere  MarkerSize=10  GraphicVisPropType=SimpleVisualProperties  GraphicDiffuseColor=[0.2314 0.2314 0.2314]  GraphicOpacity=1  GraphicSpecularColor=[0.5 0.5 0.5 1.0]  GraphicAmbientColor=[0.15 0.15 0.15 1.0]  GraphicEmissiveColor=[0.0 0.0 0.0 1.0]  GraphicShininess=75  DoExposeReferenceFrame=on  SerializedFrames=<Frames/>
  base lower : sm_lib/Body Elements/Cylindrical Solid  CylinderRadius=revCylPinDia/2  CylinderRadiusUnits=mm  CylinderLength=revCylPinLength  CylinderLengthUnits=mm  ExportEntireGeometry=off  InertiaType=CalculateFromGeometry  BasedOnType=Density  Density=1000  DensityUnits=kg/m^3  Mass=1  MassUnits=kg  CenterOfMass=[0 0 0]  CenterOfMassUnits=m  MomentsOfInertia=[1 1 1]  MomentsOfInertiaUnits=kg*m^2  ProductsOfInertia=[0 0 0]  ProductsOfInertiaUnits=kg*m^2  GraphicType=FromGeometry  MarkerShape=Sphere  MarkerSize=10  GraphicVisPropType=SimpleVisualProperties  GraphicDiffuseColor=[0.2314 0.2314 0.2314]  GraphicOpacity=1  GraphicSpecularColor=[0.5 0.5 0.5 1.0]  GraphicAmbientColor=[0.15 0.15 0.15 1.0]  GraphicEmissiveColor=[0.0 0.0 0.0 1.0]  GraphicShininess=75  DoExposeReferenceFrame=on  SerializedFrames=<Frames/>
  CylJointLow : PMIOPort  Side=Left
  CylJointTop : PMIOPort  Port=2  Side=Right
  connections:
  TF_transBaseG/RConn1 -- Subsystem/LConn1 -- base global/RConn1
  World Frame/RConn1 -- Mechanism Configuration/RConn1 -- TF_transBaseG/LConn1 -- TF_transBaseL/LConn1
  base lower/RConn1 -- CylJointLow/RConn1 -- TF_rotBaseL/RConn1
  TF_transBaseL/RConn1 -- TF_rotBaseL/LConn1
  CylJointTop/RConn1 -- Subsystem/RConn1

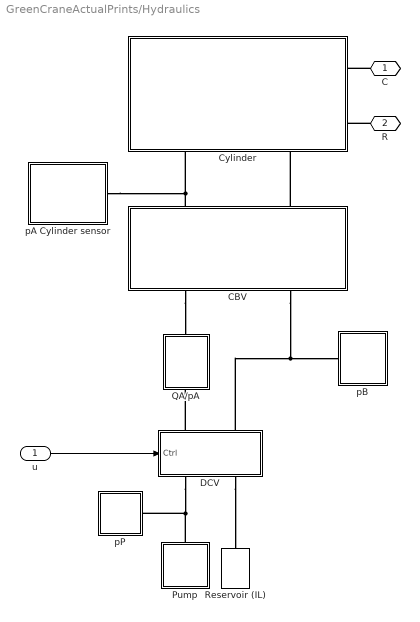
== system GreenCraneActualPrints/Hydraulics ==
  u : Inport
  CBV : Subsystem
  Cylinder : Subsystem
      settings: PortSchema="{\"entries\":[{\"content\":{\"sides\":[{\"content\":{},\"type\":\"ConnectorPlacement.EquallySpacedRectSide\",\"uuid\":\"e1757439-da3d-4938-a6aa-60b047833215\"},{\"content\":{\"connectorIds\":[\"RConn1\",\"RConn2\"],\"side\":\"RIGHT\"},\"type\":\"ConnectorPlacement.EquallySpacedRectSide\",\"uuid\":\"99876049-c36c-43ae-a9a7-33d45793de45\"},{\"content\":{\"side\":\"TOP\"},\"type\":\"ConnectorPlacement.EquallySpacedRectSide\",\"uuid\":\"2c75668b-3816-4d0f-9703-dc97a0927f4e\"},{\"content\":{\"connectorIds\":[\"RConn3\",\"RConn4\"],\"side\":\"BOTTOM\"},\"type\":\"ConnectorPlacement.EquallySpacedRectSide\",\"uuid\":\"20c5fd7e-9d5b-4b11-9210-52d97b0b3b5d\"}]},\"type\":\"ConnectorPlacement.EquallySpacedConnector\",\"uuid\":\"8c03c779-7a1d-4068-9a99-b8774a02bfc2\"}],\"packageUris\":[\"http://schema.mathworks.com/mf0/Connector/R2020b\"],\"version\":\"1.0\"}"
  DCV : Subsystem
      settings: PortSchema="{\"entries\":[{\"content\":{\"sides\":[{\"content\":{\"connectorIds\":[\"In1\"]},\"type\":\"ConnectorPlacement.EquallySpacedRectSide\",\"uuid\":\"82efbe16-358b-43f5-842f-5139282b384b\"},{\"content\":{\"side\":\"RIGHT\"},\"type\":\"ConnectorPlacement.EquallySpacedRectSide\",\"uuid\":\"01a53a89-2e01-4fc7-8dc3-3d8ddf59a6a3\"},{\"content\":{\"connectorIds\":[\"LConn1\",\"LConn2\"],\"side\":\"TOP\"},\"type\":\"ConnectorPlacement.EquallySpacedRectSide\",\"uuid\":\"a39e932d-ccaa-4d3e-8f6b-b4090f85e13b\"},{\"content\":{\"connectorIds\":[\"RConn1\",\"RConn2\"],\"side\":\"BOTTOM\"},\"type\":\"ConnectorPlacement.EquallySpacedRectSide\",\"uuid\":\"88a210a1-af22-43b5-9e88-c1c5dd6e4710\"}]},\"type\":\"ConnectorPlacement.EquallySpacedConnector\",\"uuid\":\"0289e9f8-fe04-41e6-bac5-792186d236ec\"}],\"packageUris\":[\"http://schema.mathworks.com/mf0/Connector/R2020b\"],\"version\":\"1.0\"}"
  Pump : Subsystem
      settings: PortSchema="{\"entries\":[{\"content\":{\"sides\":[{\"content\":{},\"type\":\"ConnectorPlacement.EquallySpacedRectSide\",\"uuid\":\"d756be92-1bc7-4a0a-89ff-2b4e6bfb261c\"},{\"content\":{\"side\":\"RIGHT\"},\"type\":\"ConnectorPlacement.EquallySpacedRectSide\",\"uuid\":\"fb3195af-1afb-4ef7-aeb0-1f96c2ed7014\"},{\"content\":{\"connectorIds\":[\"LConn1\"],\"side\":\"TOP\"},\"type\":\"ConnectorPlacement.EquallySpacedRectSide\",\"uuid\":\"bfa4d591-3bdc-4e9a-894e-faac675e963a\"}]},\"type\":\"ConnectorPlacement.EquallySpacedConnector\",\"uuid\":\"e539a458-eb3c-45cc-8fca-a2646cfbb4f3\"}],\"packageUris\":[\"http://schema.mathworks.com/mf0/Connector/R2020b\"],\"version\":\"1.0\"}"
  QA/pA : Subsystem
      settings: PortSchema="{\"entries\":[{\"content\":{\"sides\":[{\"content\":{},\"type\":\"ConnectorPlacement.EquallySpacedRectSide\",\"uuid\":\"528edc0f-4a4d-4637-aeac-ce7d4705c794\"},{\"content\":{\"side\":\"RIGHT\"},\"type\":\"ConnectorPlacement.EquallySpacedRectSide\",\"uuid\":\"1212f0bf-cd1d-49c9-8d64-2c2fa0f26d5e\"},{\"content\":{\"connectorIds\":[\"LConn1\"],\"side\":\"TOP\"},\"type\":\"ConnectorPlacement.EquallySpacedRectSide\",\"uuid\":\"19f63e16-fedb-4531-944d-7dd5973f4706\"},{\"content\":{\"connectorIds\":[\"RConn1\"],\"side\":\"BOTTOM\"},\"type\":\"ConnectorPlacement.EquallySpacedRectSide\",\"uuid\":\"97241fcf-5bdd-4391-919c-4f6f215da4de\"}]},\"type\":\"ConnectorPlacement.EquallySpacedConnector\",\"uuid\":\"f2c4e0d1-02bc-4c64-99f2-26e77e9ed48e\"}],\"packageUris\":[\"http://schema.mathworks.com/mf0/Connector/R2020b\"],\"version\":\"1.0\"}"
  Reservoir (IL) : fl_lib/Isothermal Liquid/Elements/Reservoir (IL)  reservoir_type=foundation.enum.constant_controlled.constant  pressure_spec=foundation.enum.pressure_spec.atmospheric  reservoir_pressure=0.101325 MPa
  pA Cylinder sensor : Subsystem
  pB : Subsystem
  pP : Subsystem
  C : PMIOPort  Side=Right
  R : PMIOPort  Port=2  Side=Right
  wires:
  u/1 -> DCV/1(Ctrl)
  connections:
  CBV/LConn2 -- DCV/LConn2 -- pB/LConn1
  Pump/LConn1 -- DCV/RConn1 -- pP/LConn1
  pA Cylinder sensor/LConn1 -- CBV/RConn1 -- Cylinder/RConn3
  C/RConn1 -- Cylinder/RConn1
  R/RConn1 -- Cylinder/RConn2
  CBV/LConn1 -- QA/pA/LConn1
  DCV/LConn1 -- QA/pA/RConn1
  DCV/RConn2 -- Reservoir (IL)/LConn1
  CBV/RConn2 -- Cylinder/RConn4

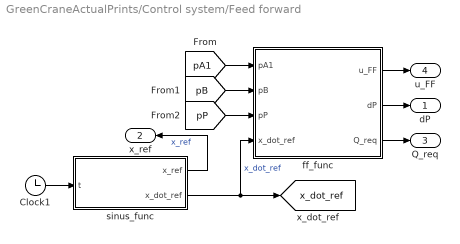
== system GreenCraneActualPrints/Control system/Feed forward ==
  Clock1 : Clock
  ff_func : MATLAB Function  TreatAsAtomicUnit=on
  sinus_func : MATLAB Function  TreatAsAtomicUnit=on
  dP : Outport
  x_ref : Outport  Port=2
  Q_req : Outport  Port=3
  u_FF : Outport  Port=4
  tag scope: x_dot_ref=global
  wires:
  Clock1/1 -> sinus_func/1(t)
  [pA1] -> ff_func/1(pA1)
  [pP] -> ff_func/3(pP)
  [pB] -> ff_func/2(pB)
  ff_func/2(dP) -> dP/1
  ff_func/3(Q_req) -> Q_req/1
  ff_func/1(u_FF) -> u_FF/1
  sinus_func/2(x_dot_ref) -> ff_func/4(x_dot_ref), [x_dot_ref]  "x_dot_ref"
  sinus_func/1(x_ref) -> x_ref/1  "x_ref"

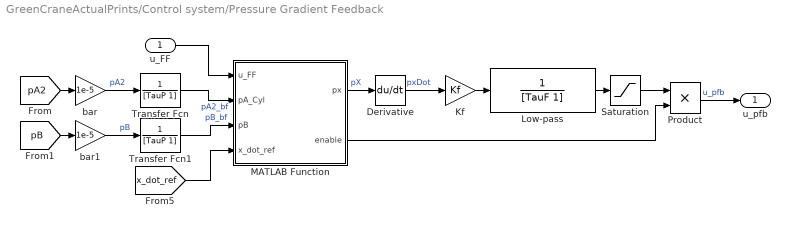
== system GreenCraneActualPrints/Control system/Pressure Gradient Feedback ==
  u_FF : Inport
  Derivative : Derivative
  Kf : Gain  Gain=Kf
  Low-pass : TransferFcn  Denominator=[TauF 1]
  MATLAB Function : MATLAB Function  TreatAsAtomicUnit=on
  Product : Product
  Saturation : Saturate  UpperLimit=0.1  LowerLimit=-0.1
  Transfer Fcn : TransferFcn  Denominator=[TauP 1]
  Transfer Fcn1 : TransferFcn  Denominator=[TauP 1]
  bar : Gain  Gain=1e-5
  bar1 : Gain  Gain=1e-5
  u_pfb : Outport
  wires:
  MATLAB Function/1(px) -> Derivative/1  "pX"
  Derivative/1 -> Kf/1  "pxDot"
  [x_dot_ref] -> MATLAB Function/4(x_dot_ref)
  u_FF/1 -> MATLAB Function/1(u_FF)
  [pA2] -> bar/1
  bar/1 -> Transfer Fcn/1  "pA2"
  Kf/1 -> Low-pass/1
  Low-pass/1 -> Saturation/1
  [pB] -> bar1/1
  bar1/1 -> Transfer Fcn1/1  "pB"
  Transfer Fcn/1 -> MATLAB Function/2(pA_Cyl)  "pA2_bf"
  Transfer Fcn1/1 -> MATLAB Function/3(pB)  "pB_bf"
  Product/1 -> u_pfb/1  "u_pfb"
  Saturation/1 -> Product/1
  MATLAB Function/2(enable) -> Product/2
